simulink model "lab01"  (R2020b)
settings: Solver=VariableStepAuto  StartTime=0.0  StopTime=10.0  RelTol=1e-3
settings Model: Creator=karth  LastModifiedBy=karth

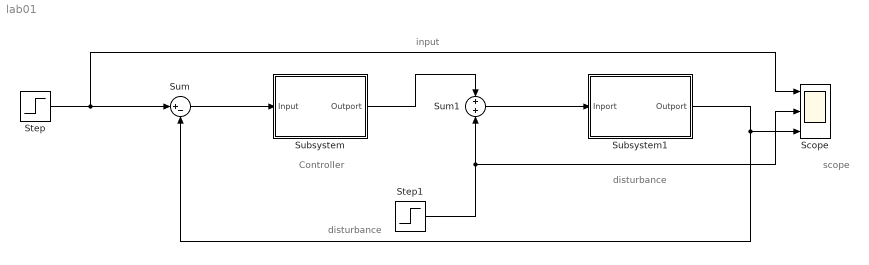
== system lab01 ==
  note: disturbance
  note: scope
  note: input
  note: Controller
  note: disturbance
  Scope : Scope  NumInputPorts=3
  Step : Step  SampleTime=0
  Step1 : Step  SampleTime=0
  Subsystem : Subsystem
  Subsystem1 : Subsystem
  Sum : Sum  Inputs=|+-
  Sum1 : Sum
  wires:
  Step/1 -> Scope/1, Sum/1
  Sum/1 -> Subsystem/1(Input)
  Subsystem/1(Outport) -> Sum1/1
  Sum1/1 -> Subsystem1/1(Inport)
  Step1/1 -> Scope/2, Sum1/2
  Subsystem1/1(Outport) -> Sum/2, Scope/3

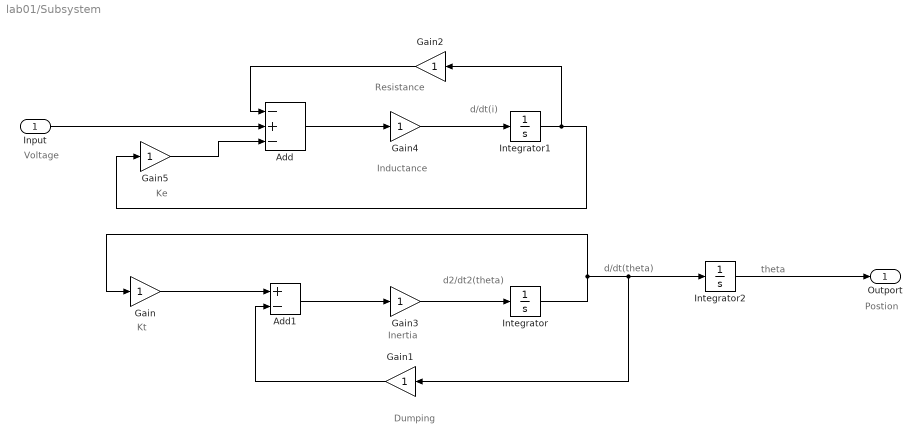
== system lab01/Subsystem ==
  note: Postion
  note: theta
  note: d2/dt2(theta)
  note: Dumping
  note: Inertia
  note: d/dt(i)
  note: Inductance
  note: Resistance
  note: Kt
  note: Ke
  note: Voltage
  note: d/dt(theta)
  Input : Inport
  Add : Sum  Inputs=-+-
  Add1 : Sum  Inputs=+-
  Gain{,1..5} (6 alike) : Gain
  Integrator : Integrator
  Integrator1 : Integrator
  Integrator2 : Integrator
  Outport : Outport
  wires:
  Gain3/1 -> Integrator/1
  Gain/1 -> Add1/1
  Gain4/1 -> Integrator1/1
  Integrator/1 -> Gain1/1, Integrator2/1, Gain/1
  Add/1 -> Gain4/1
  Integrator2/1 -> Outport/1
  Integrator1/1 -> Gain2/1, Gain5/1
  Gain2/1 -> Add/1
  Gain5/1 -> Add/3
  Add1/1 -> Gain3/1
  Gain1/1 -> Add1/2
  Input/1 -> Add/2

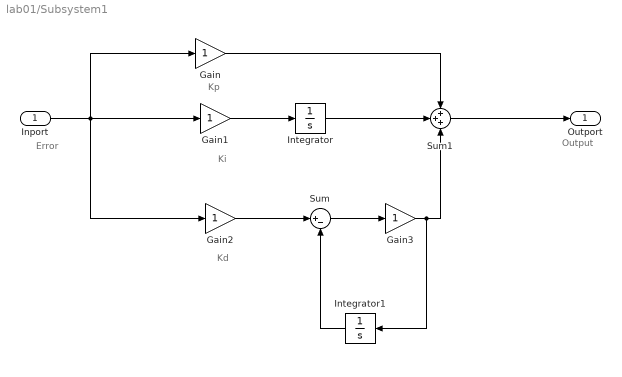
== system lab01/Subsystem1 ==
  note: Kd
  note: Ki
  note: Kp
  note: Error
  note: Output
  Inport : Inport
  Gain{,1..3} (4 alike) : Gain
  Integrator : Integrator
  Integrator1 : Integrator
  Sum : Sum  Inputs=|+-
  Sum1 : Sum  Inputs=+++
  Outport : Outport
  wires:
  Sum/1 -> Gain3/1
  Inport/1 -> Gain2/1, Gain/1, Gain1/1
  Integrator/1 -> Sum1/2
  Gain1/1 -> Integrator/1
  Gain/1 -> Sum1/1
  Integrator1/1 -> Sum/2
  Gain3/1 -> Integrator1/1, Sum1/3
  Sum1/1 -> Outport/1
  Gain2/1 -> Sum/1
